simulink model "asbCubeSat"  (R2023b)
settings: Solver=FixedStepAuto  StartTime=0.0  StopTime=43200  FixedStep=CubeSatTimeStep  MaxStep=10  MinStep=0.01  RelTol=1e-7  AbsTol=1e-7  EnableMultiTasking=on
PreLoadFcn:
  | if ~builtin('license','test','Virtual_Reality_Toolbox')
  |     dd = Simulink.data.dictionary.open('asbCubeSatModelData.sldd');
  |     ddSect = getSection(dd, 'Design Data');
  |     assignin(ddSect,'variantVisualization',0)
  | end
InitFcn:
  | temp_dd = Simulink.data.dictionary.open('asbCubeSatModelData.sldd');
  | temp_ddSect = getSection(temp_dd, 'Design Data');
  | if evalin(temp_ddSect, 'variantVisualization == 1')
  |     if ~builtin('license','checkout','Virtual_Reality_Toolbox')
  |         error(message('aeroblks_cubesat:cubesat:licenseFailAnim'));
  |     end
  | end
  | clear temp_dd temp_ddSect;
undefined symbols (not defined in the file): actuator, asbCubeSatEnvironmentLib, CubeSatTimeStep, Enviroment, initCond, WMM2020
libraries: aerolibutil x16, sharedutil x4, aerolibconvert2 x4, matrix_library x3, aerolibattitudesys x2, simulink_extras x2, sharedtransform x2, aerolibgravity2 x1, SignalEditorBlockLib x1, aerolibtransform2 x1, asbCubeSatFSWLib x1, aerolibobsolete x1
settings Model: RequirementInfo={} %GIDa_aedc6be2_fb6a_446c_8c25_10b8bc9db182  DataDictionary=asbCubeSatModelData.sldd  SnapshotInterval=1  Creator=The MathWorks, Inc.  LastModifiedBy=Adin Sacho-Tanzer
settings SolverCC: AlgebraicLoopSolver=TrustRegion  MaxZcPerStep=1
settings DataIOCC: LimitDataPoints=on  SaveFormat=Array  SaveOutput=off  DSMLogging=off  SaveTime=off  ReturnWorkspaceOutputs=off
settings OptimizationCC: DefaultParameterBehavior=Inlined  OptimizeBlockIOStorage=off  BufferReuse=off  GlobalBufferReuse=off  ExpressionFolding=off  ExpressionDepthLimit=2147483647  LocalBlockOutputs=off  InitFltsAndDblsToZero=on  LifeSpan=inf  OptimizeDataStoreBuffers=off  BusAssignmentInplaceUpdate=off
settings DebuggingCC: SignalResolutionControl=TryResolveAllWithWarning  MultiTaskDSMMsg=warning  MultiTaskCondExecSysMsg=none  UnconnectedInputMsg=warning  UnconnectedOutputMsg=warning  UnconnectedLineMsg=warning  AssertControl=DisableAll  ModelReferenceExtraNoncontSigs=warning  StateNameClashWarn=warning  PregeneratedLibrarySubsystemCodeDiagnostic=none  SFUnexpectedBacktrackingDiag=warning  SFNoUnconditionalDefaultTransitionDiag=warning  SFExecutionAtInitializationDiag=none  ArithmeticOperatorsInVariantConditions=warning
settings HardwareCC: ProdBitPerPointer=32  ProdBitPerSizeT=32  ProdBitPerPtrDiffT=32  ProdLargestAtomicFloat=None  ProdIntDivRoundTo=Undefined  ProdEndianess=Unspecified  ProdWordSize=32  ProdHWDeviceType=32-bit Generic
settings ModelReferenceCC: UpdateModelReferenceTargets=IfOutOfDate  EnableRefExpFcnMdlSchedulingChecks=on  ModelReferenceMinAlgLoopOccurrences=on  PropagateSignalLabelsOutOfModel=off
settings SFSimCC: SimUseLocalCustomCode=off
settings RTWCC: RTWUseLocalCustomCode=off  DLArmComputeVersion=19.05
settings CodeAppCC: StateflowObjectComments=on
settings GRTTargetCC: TargetFcnLib=ansi_tfl_tmw.mat  TargetLangStandard=C89/C90 (ANSI)  CombineOutputUpdateFcns=off  GRTInterface=on
settings ConfigComp: CovMetricSettings=dw  CovSaveCumulativeToWorkspaceVar=on  CovSaveSingleToWorkspaceVar=on  CovExternalEMLEnable=off

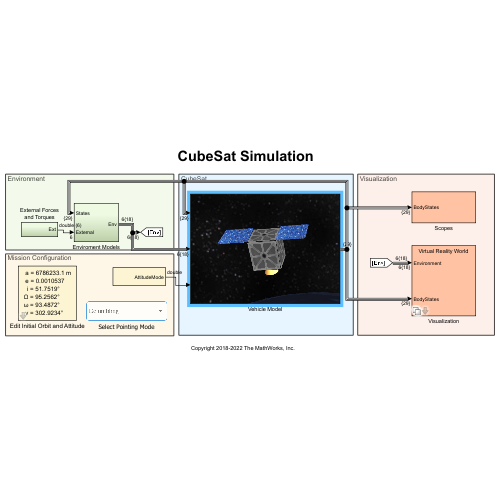
[thumbnail: Simulink's stored preview of the top-level diagram]
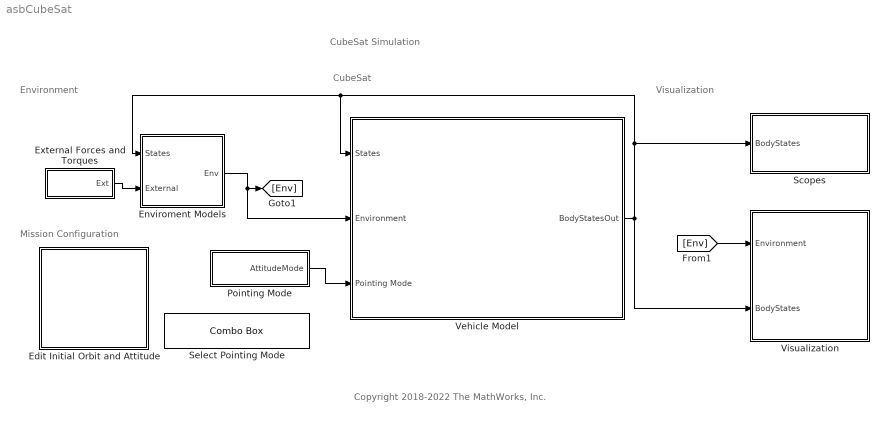
== system asbCubeSat ==
  note: Visualization
  note: CubeSat
  note: Environment
  note: Copyright 2018-2022 The MathWorks, Inc.
  note: CubeSat Simulation
  note: Mission Configuration
  Edit Initial Orbit and Attitude : Subsystem  mask(CubeSat Initial Conditions){sim_t0=2458488, epoch=2451545, method=Keplerian Orbital Elements, a=6786233.13, ecc=0.0010537, incl=51.7519, omega=95.2562, argp=93.4872, nu=302.9234, truelon=0, arglat=0, lonper=0, r_eci=[-2981784.257 5207055.9381 3161595.3068], v_eci=[-3384.4834 -4887.7595 4843.4609], r_ecef=[-5762650.9114 -1682704.282 3156028.2879], v_ecef=[3832.57 -4024.9014 4837.4311], lla=[27.88080034 -163.722102 408851.6223], v_ned=[5468.7396 4937.8129 -7.4627367], euler=[33.9 -5.91 9.88], pqr=[10 10 0]}
      mask prompts: sim_t0 "spacecraft:cubesat:StartDate"; epoch "spacecraft:cubesat:ECIEpoch"; method "spacecraft:cubesat:InputMethod"; a "spacecraft:cubesat:SemiMajorAxis"; ecc "spacecraft:cubesat:Eccentricity"; incl "spacecraft:cubesat:Inclination"; omega "spacecraft:cubesat:RAAN"; argp "spacecraft:cubesat:ArgP"; nu "spacecraft:cubesat:TrueAnomaly"; truelon "spacecraft:cubesat:TrueLon"; arglat "spacecraft:cubesat:ArgLat"; lonper "spacecraft:cubesat:LonPer"; r_eci "spacecraft:cubesat:ECIPos"; v_eci "spacecraft:cubesat:ECIVel"; r_ecef "spacecraft:cubesat:ECEFPos"; v_ecef "spacecraft:cubesat:ECEFVel"; lla "spacecraft:cubesat:LLA"; v_ned "spacecraft:cubesat:NEDVel"; euler "spacecraft:cubesat:Euler"; pqr "spacecraft:cubesat:BodyAngRates"
      mask help: spacecraft:cubesat:InitCondBlockDesc
      mask init:
      | initCond = cubeSatCallback(gcb, 'computeIC', method, sim_t0, epoch, a, ecc, incl,...
      |     omega, argp, nu, truelon, arglat, lonper, r_eci, v_eci, r_ecef, v_ecef, lla,...
      |     v_ned, euler, pqr);
      mask TypeOptions method: spacecraft:cubesat:InputKeplerian | spacecraft:cubesat:InputECI | spacecraft:cubesat:InputECEF | spacecraft:cubesat:InputLLANED
      mask Callback method: cubeSatCallback(gcb, 'handleMethod');
      mask Callback ecc: cubeSatCallback(gcb, 'handleCircularOrbit');
      mask Callback incl: cubeSatCallback(gcb, 'handleCircularOrbit');
      mask DialogControl sim_t0 Prompt: Start date [Julian date]:
      mask DialogControl sim_t0 Tooltip: spacecraft:spacecraft:StartDateTT
      mask DialogControl icTab Prompt: spacecraft:cubesat:InitCond
      mask DialogControl epoch Prompt: Epoch of ECI frame [Julian date]:
      mask DialogControl epoch Tooltip: spacecraft:cubesat:ECIEpochTT
      mask DialogControl Container9 Prompt: spacecraft:cubesat:InitCondOrbit
      mask DialogControl method Prompt: Input method:
      mask DialogControl method Tooltip: spacecraft:cubesat:InputMethodTT
      mask DialogControl a Prompt: Semi-major axis [m]:
      mask DialogControl a Tooltip: spacecraft:cubesat:SemiMajorAxisTT
      mask DialogControl ecc Prompt: Eccentricity:
      mask DialogControl ecc Tooltip: spacecraft:cubesat:EccentricityTT
      mask DialogControl incl Prompt: Inclination [deg]:
      mask DialogControl incl Tooltip: spacecraft:cubesat:InclinationTT
      mask DialogControl omega Prompt: Right ascension of the ascending node [deg]:
      mask DialogControl omega Tooltip: spacecraft:cubesat:RAANTT
      mask DialogControl argp Prompt: Argument of periapsis [deg]:
      mask DialogControl argp Tooltip: spacecraft:cubesat:ArgPTT
      mask DialogControl nu Prompt: True anomaly [deg]:
      mask DialogControl nu Tooltip: spacecraft:cubesat:TrueAnomalyTT
      mask DialogControl truelon Prompt: True longitude [deg] (circular equatorial):
      mask DialogControl truelon Tooltip: spacecraft:cubesat:TrueLonTT
      mask DialogControl arglat Prompt: Argument of latitude [deg] (circular inclined):
      mask DialogControl arglat Tooltip: spacecraft:cubesat:ArgLatTT
      mask DialogControl lonper Prompt: Longitude of periapsis [deg] (elliptical equatorial):
      mask DialogControl lonper Tooltip: spacecraft:cubesat:LonPerTT
      mask DialogControl r_eci Prompt: ECI position vector [m]:
      mask DialogControl r_eci Tooltip: spacecraft:cubesat:ECIPosTT
      mask DialogControl v_eci Prompt: ECI velocity vector [m/s]:
      mask DialogControl v_eci Tooltip: spacecraft:cubesat:ECIVelTT
      mask DialogControl r_ecef Prompt: ECEF position vector [m]:
      mask DialogControl r_ecef Tooltip: spacecraft:cubesat:ECEFPosTT
      mask DialogControl v_ecef Prompt: ECEF velocity vector [m/s]:
      mask DialogControl v_ecef Tooltip: spacecraft:cubesat:ECEFVelTT
      mask DialogControl lla Prompt: Geodetic latitude, longitude, altitude [deg, deg, m]:
      mask DialogControl lla Tooltip: spacecraft:cubesat:LLATT
      mask DialogControl v_ned Prompt: NED velocity vector [m/s]:
      mask DialogControl v_ned Tooltip: spacecraft:cubesat:NEDVelTT
      mask DialogControl Container11 Prompt: spacecraft:cubesat:InitCondAttitude
      mask DialogControl euler Prompt: Initial Euler angles (roll, pitch, yaw) [deg]:
      mask DialogControl euler Tooltip: spacecraft:cubesat:EulerTT
      mask DialogControl pqr Prompt: Initial body angular rates [deg/s]:
      mask DialogControl pqr Tooltip: spacecraft:cubesat:BodyAngRatesTT
      mask Display:
      | text(.1, .9, [' a = ' sprintf('%.1f', str2double(get_param(gcb, 'a'))) ' m'],'horizontalAlignment','left','texmode','on');
      | text(.1, .75, [' e = ' get_param(gcb, 'ecc')],'horizontalAlignment','left','texmode', 'on')
      | text(.1, .6, ['  i = ' get_param(gcb, 'incl') '\circ'],'horizontalAlignment','left','texmode', 'on')
      | text(.1, .45, ['\Omega = ' get_param(gcb, 'omega') '\circ'],'horizontalAlignment','left','texmode', 'on')
      | text(.1, .3, ['\omega = ' get_param(gcb, 'argp') '\circ'],'horizontalAlignment','left','texmode', 'on')
      | text(.1, .15, [' \nu = ' get_param(gcb, 'nu') '\circ'],'horizontalAlignment','left','texmode', 'on')
  Enviroment Models : Subsystem  AncestorBlock=asbCubeSatEnvironmentLib/Enviroment
  "External Forces and Torques " : Subsystem
  Pointing Mode : Subsystem
  Scopes : Subsystem  VariantControl=visOff
  Select Pointing Mode : ComboBox  LabelPosition=Hide  SelectedLabel=Detumbling
      settings: Values={{'Standby', 'Nadir Pointing (Earth)', 'Sun Tracking', 'Custom Schedule', 'Detumbling'}, [0 1 2 3 4]}
  Vehicle Model : Subsystem
      mask Display: image('CubeSatVehicle.PNG');
  Visualization : Subsystem  Variant=on  mask(Set Animation Properties){visSampleTime=5, cubesatSize=2e5, showAntenna=on, antennaHeight=1e6, antennaHalfAngle=25}
      mask prompts: visSampleTime "spacecraft:cubesat:AnimSampleTime"; cubesatSize "spacecraft:cubesat:MdlSize"; showAntenna "spacecraft:cubesat:ShowCone"; antennaHeight "spacecraft:cubesat:ConeHeight"; antennaHalfAngle "spacecraft:cubesat:ConeAngle"
      mask help: spacecraft:cubesat:VisBlockDesc
      mask Callback showAntenna:
      | if builtin('license','test','Virtual_Reality_Toolbox')
      | 
      |     enable = get_param(gcb,'MaskEnables');
      |     if strcmp(get_param(gcb, 'showAntenna'), 'off')
      |         enable(4:5) = {'off'};
      |     else
      |         enable(4:5) = {'on'};
      |     end
      |     set_param(gcb,'MaskEnables', enable);
      |     clear enable
      | end
      mask DialogControl vrOpenBtn Prompt: spacecraft:cubesat:AnimOpenBtn
      mask DialogControl vrOpenBtn Callback:
      | if builtin('license','checkout','Virtual_Reality_Toolbox')
      |     vrmfunc('FnOpen',getSimulinkBlockHandle([gcb '/Virtual Reality World/VR Sink']));
      | end
      mask DialogControl visSampleTime Prompt: Animation refresh rate:
      mask DialogControl visSampleTime Tooltip: spacecraft:cubesat:AnimSampleTimeTT
      mask DialogControl cubesatSize Prompt: CubeSat display size [m]:
      mask DialogControl cubesatSize Tooltip: spacecraft:cubesat:MdlSizeTT
      mask DialogControl Container3 Prompt: spacecraft:cubesat:AntennaPropArea
      mask DialogControl showAntenna Prompt: Show antenna cone in animation
      mask DialogControl showAntenna Tooltip: spacecraft:cubesat:ShowConeTT
      mask DialogControl antennaHeight Prompt: Antenna cone height [m]:
      mask DialogControl antennaHeight Tooltip: spacecraft:cubesat:ConeHeightTT
      mask DialogControl antennaHalfAngle Prompt: Antenna cone half angle [deg]:
      mask DialogControl antennaHalfAngle Tooltip: spacecraft:cubesat:ConeAngleTT
  wires:
  Enviroment Models/1(Env) -> Vehicle Model/2(Environment), [Env]
  "External Forces and Torques "/1(Ext) -> Enviroment Models/2(External)
  Pointing Mode/1(AttitudeMode) -> Vehicle Model/3(Pointing Mode)
  [Env] -> Visualization/1(Environment)
  Vehicle Model/1(BodyStatesOut) -> Visualization/2(BodyStates), Vehicle Model/1(States), Enviroment Models/1(States), Scopes/1(BodyStates)

== system asbCubeSat/Edit Initial Orbit and Attitude ==

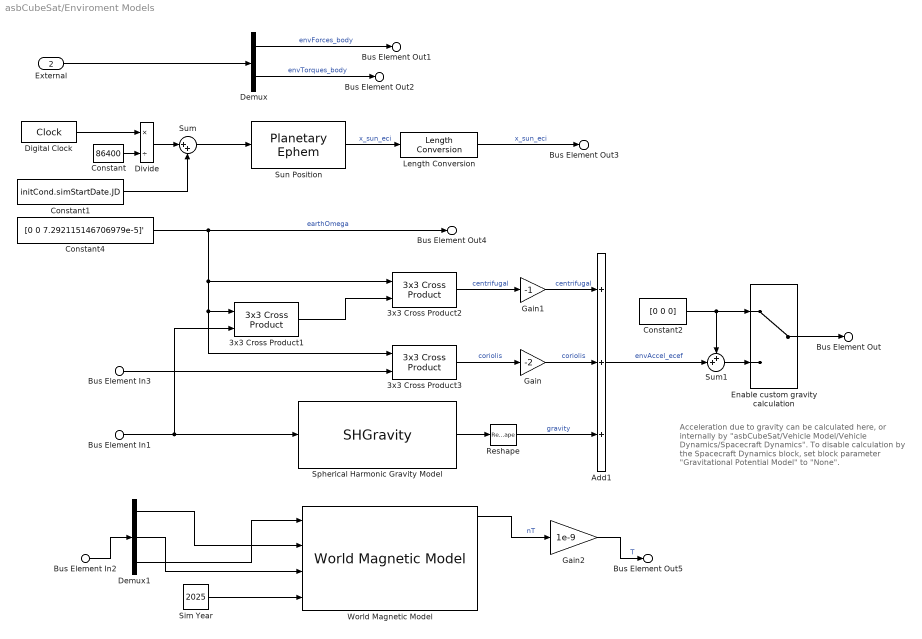
== system asbCubeSat/Enviroment Models ==
  note: Acceleration due to gravity can be calculated here, or internally by "asbCubeSat/Vehicle Model/Vehicle Dynamics/Spacecraft Dynamics". To disable calculation by the Spacecraft Dynamics block, set block parameter "Gravitational Potential Model" to "None".
  Bus Element In1 : Inport  PortName=States  Element=X_ecef
  Bus Element In3 : Inport  PortName=States  Element=V_ecef
  Bus Element In2 : Inport  PortName=States  Element=LatLonAlt
  External : Inport  RequirementInfo={} %GIDa_966e36cb_16b5_4872_900e_7ca1bd630c23  Port=2
  3x3 Cross Product1 : sharedutil/3x3 Cross Product  aMode=aMode
  3x3 Cross Product2 : sharedutil/3x3 Cross Product  aMode=aMode
  3x3 Cross Product3 : sharedutil/3x3 Cross Product  aMode=aMode
  Add1 : Sum  RequirementInfo={} %GIDa_b8d2c483_28a5_4509_a823_93e900185cc4  Inputs=+++
  Constant : Constant  Value=86400
  Constant1 : Constant  RequirementInfo={} %GIDa_d3dce1ea_7a4c_4489_9b49_860fce94c68a  Value=initCond.simStartDate.JD
  Constant2 : Constant  RequirementInfo={} %GIDa_bd077cfd_f306_41c3_b781_8f19467a1c05  Value=[0 0 0]
  Constant4 : Constant  Value=[0 0 7.292115146706979e-5]'
  Demux : Demux  RequirementInfo={} %GIDa_25e02362_af2f_4200_81e6_6d7271b48bfe  Outputs=2
  Demux1 : Demux  Outputs=3
  Digital Clock : DigitalClock  SampleTime=CubeSatTimeStep
  Divide : Product  Inputs=*/
  Enable custom gravity calculation : ManualSwitch
  Gain : Gain  Gain=-2
  Gain1 : Gain  Gain=-1
  Gain2 : Gain  Gain=1e-9
  Length Conversion : aerolibconvert2/Length Conversion  IU=km  OU=m
  Reshape : Reshape
  Sim Year : Constant  Value=2025
  Spherical Harmonic Gravity Model : SHGravity  RequirementInfo={} %GIDa_e6b23945_77d7_4eed_b23b_331bed44acc0  degree=20  datafile='aerogmm2b.mat'
  Sum : Sum  Inputs=|++
  Sum1 : Sum  Inputs=++|
  Sun Position : PlanetaryEphem  ephemerisModel=DE421  target=Sun  outputVelocity=off
  World Magnetic Model : aerolibgravity2/World Magnetic Model  model=WMM2020 (2020-2025)  customFile='WMM2020.COF'  units=Metric (MKS)  time_in=on  month=January  day=1  year=2020  action=Error  h_out=on  dec_out=on  inc_out=on  ti_out=on
  Bus Element Out : Outport  VectorParamsAs1DForOutWhenUnconnected=off  PortName=Env  Element=envAccel_ecef
  Bus Element Out1 : Outport  VectorParamsAs1DForOutWhenUnconnected=off  PortName=Env  Element=envForces_body
  Bus Element Out2 : Outport  VectorParamsAs1DForOutWhenUnconnected=off  PortName=Env  Element=envTorques_body
  Bus Element Out3 : Outport  VectorParamsAs1DForOutWhenUnconnected=off  PortName=Env  Element=x_sun_eci
  Bus Element Out4 : Outport  VectorParamsAs1DForOutWhenUnconnected=off  PortName=Env  Element=earthAngRate
  Bus Element Out5 : Outport  VectorParamsAs1DForOutWhenUnconnected=off  PortName=Env  Element=mag_NED
  wires:
  Sum1/1 -> Enable custom gravity calculation/2
  Enable custom gravity calculation/1 -> Bus Element Out/1
  Constant2/1 -> Enable custom gravity calculation/1, Sum1/1
  Gain/1 -> Add1/2  "coriolis"
  Gain1/1 -> Add1/1  "centrifugal"
  3x3 Cross Product2/1 -> Gain1/1  "centrifugal"
  3x3 Cross Product3/1 -> Gain/1  "coriolis"
  Bus Element In3/1 -> 3x3 Cross Product3/2
  3x3 Cross Product1/1 -> 3x3 Cross Product2/2
  Reshape/1 -> Add1/3  "gravity"
  Constant1/1 -> Sum/2
  Divide/1 -> Sum/1
  Constant/1 -> Divide/2
  Length Conversion/1 -> Bus Element Out3/1  "x_sun_eci"
  Constant4/1 -> 3x3 Cross Product2/1, 3x3 Cross Product1/1, 3x3 Cross Product3/1, Bus Element Out4/1  "earthOmega"
  Sun Position/1 -> Length Conversion/1  "x_sun_eci"
  Digital Clock/1 -> Divide/1
  Sum/1 -> Sun Position/1
  Spherical Harmonic Gravity Model/1 -> Reshape/1
  External/1 -> Demux/1
  Demux/2 -> Bus Element Out2/1  "envTorques_body"
  Add1/1 -> Sum1/2  "envAccel_ecef"
  Demux/1 -> Bus Element Out1/1  "envForces_body"
  Bus Element In1/1 -> Spherical Harmonic Gravity Model/1, 3x3 Cross Product1/2
  Bus Element In2/1 -> Demux1/1
  Demux1/1 -> World Magnetic Model/2
  Demux1/3 -> World Magnetic Model/1
  Demux1/2 -> World Magnetic Model/3
  Sim Year/1 -> World Magnetic Model/4
  World Magnetic Model/1 -> Gain2/1  "nT"
  Gain2/1 -> Bus Element Out5/1  "T"

== system asbCubeSat/External Forces and Torques  ==
  Forces_Body : Constant  Value=[0 0 0]
  Mux : Mux  RequirementInfo={} %GIDa_ef4ca723_4eef_40f8_bb1e_99de60d2b248  Inputs=2
  Torques_Body : Constant  Value=[0 0 0]
  Ext : Outport  RequirementInfo={} %GIDa_0f078eca_6127_499d_b81c_658503a40261  VectorParamsAs1DForOutWhenUnconnected=off
  wires:
  Forces_Body/1 -> Mux/1
  Torques_Body/1 -> Mux/2
  Mux/1 -> Ext/1

== system asbCubeSat/Pointing Mode ==
  note: Modes:
      | 0 = Off
      | 1 = Earth (Nadir)
      | 2 = Sun
  Mode : Constant  Value=4  SampleTime=-1
  Multiport Switch : MultiPortSwitch  DataPortOrder=Specify indices  DataPortIndices={3, [0,1,2]}  DiagnosticForDefault=None  SaturateOnIntegerOverflow=off  InputSameDT=off
  Signal Editor : SignalEditorBlockLib/Signal Editor  FileName=SignalEditorPointing.mat  ActiveScenario=PointingScenario  ActiveSignal=PointingMode  IsBus=off  OutputBusObjectStr=Bus: BusObject  SampleTime=0  Interpolate=off  ZeroCross=off  OutputAfterFinalValue=Setting to zero  Unit=inherit  PreserveSignalName=on  ApplySigPropsToAllScenarios=on  ApplySigPropsToAllSignals=off
  AttitudeMode : Outport  VectorParamsAs1DForOutWhenUnconnected=off
  wires:
  Signal Editor/1 -> Multiport Switch/2
  Mode/1 -> Multiport Switch/1, Multiport Switch/3
  Multiport Switch/1 -> AttitudeMode/1

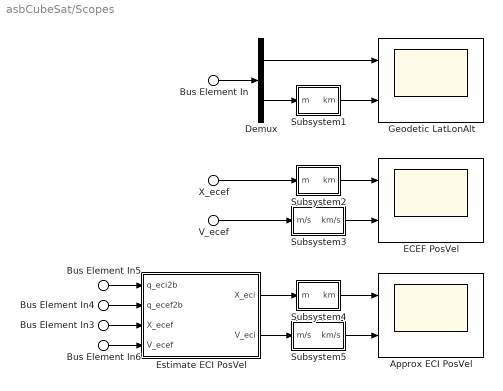
== system asbCubeSat/Scopes ==
  Bus Element In : Inport  PortName=BodyStates  Element=LatLonAlt
  X_ecef : Inport  PortName=BodyStates  Element=X_ecef
  Bus Element In3 : Inport  PortName=BodyStates  Element=X_ecef
  V_ecef : Inport  PortName=BodyStates  Element=V_ecef
  Bus Element In6 : Inport  PortName=BodyStates  Element=V_ecef
  Bus Element In4 : Inport  PortName=BodyStates  Element=q_ecef2b
  Bus Element In5 : Inport  PortName=BodyStates  Element=q_eci2b
  Approx ECI PosVel : Scope  NumInputPorts=2
  Demux : Demux  Outputs=[2 1]
  ECEF PosVel : Scope  NumInputPorts=2
  Estimate ECI PosVel : Subsystem
  Geodetic LatLonAlt : Scope  NumInputPorts=2
  Subsystem1 : Subsystem
  Subsystem2 : Subsystem
  Subsystem3 : Subsystem
  Subsystem4 : Subsystem
  Subsystem5 : Subsystem
  wires:
  Bus Element In/1 -> Demux/1
  Demux/1 -> Geodetic LatLonAlt/1
  Demux/2 -> Subsystem1/1(m)
  X_ecef/1 -> Subsystem2/1(m)
  V_ecef/1 -> Subsystem3/1(m/s)
  Estimate ECI PosVel/1(X_eci) -> Subsystem4/1(m)
  Estimate ECI PosVel/2(V_eci) -> Subsystem5/1(m/s)
  Bus Element In5/1 -> Estimate ECI PosVel/1(q_eci2b)
  Bus Element In4/1 -> Estimate ECI PosVel/2(q_ecef2b)
  Bus Element In3/1 -> Estimate ECI PosVel/3(X_ecef)
  Bus Element In6/1 -> Estimate ECI PosVel/4(V_ecef)
  Subsystem1/1(km) -> Geodetic LatLonAlt/2
  Subsystem2/1(km) -> ECEF PosVel/1
  Subsystem3/1(km/s) -> ECEF PosVel/2
  Subsystem4/1(km) -> Approx ECI PosVel/1
  Subsystem5/1(km/s) -> Approx ECI PosVel/2

== system asbCubeSat/Vehicle Model ==
  note: Flight Software
  note: Plant Model
  States : Inport
  Environment : Inport  Port=2
  Pointing Mode : Inport  Port=3
  Vehicle Control Actuators : Subsystem  AncestorBlock=asbCubeSatActuatorsLib/Vehicle Control Actuators
  Vehicle Control Sensors : Subsystem  AncestorBlock=asbCubeSatSensorsLib/Vehicle Control Sensors
  Vehicle Dynamics : Subsystem  AncestorBlock=asbCubeSatDynamicsLib/Vehicle Dynamics
  Vehicle Flight Software : asbCubeSatFSWLib/Vehicle Flight Software  SystemSampleTime=-1  VariantActivationTime=update diagram  AllowFlexibleInterface=on  Latency=0  AutoFrameSizeCalculation=off
  BodyStatesOut : Outport  OutDataTypeStr=Bus: StatesOutBus  VectorParamsAs1DForOutWhenUnconnected=off
  wires:
  Vehicle Dynamics/1(StatesOut) -> Vehicle Control Sensors/1(StatesOut), BodyStatesOut/1
  Pointing Mode/1 -> Vehicle Flight Software/1
  Vehicle Control Sensors/1(SensorsOut) -> Vehicle Flight Software/3
  Vehicle Control Actuators/1(" Forces") -> Vehicle Dynamics/1(Forces)
  Vehicle Control Actuators/2(" Torques") -> Vehicle Dynamics/2(Moments)
  Vehicle Flight Software/1 -> Vehicle Control Actuators/1(ActuatorCmds)
  Environment/1 -> Vehicle Control Actuators/2(Environment), Vehicle Dynamics/3(Env), Vehicle Flight Software/2
  States/1 -> Vehicle Control Actuators/3(States)

== system asbCubeSat/Visualization ==
  Environment : Inport
  BodyStates : Inport  RequirementInfo={} %GIDa_d1e0371a_f352_4707_a071_6ff04189e700  Port=2
  No Visualization : Subsystem  VariantControl=visOff
  Virtual Reality World : Subsystem  VariantControl=visSL3D

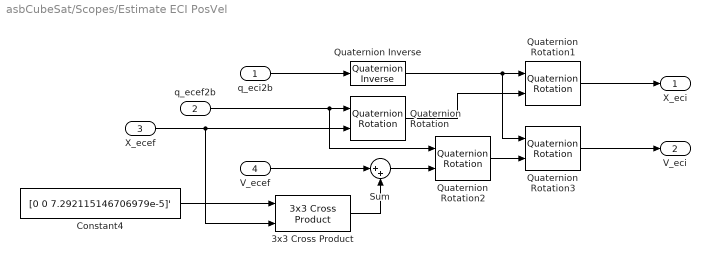
== system asbCubeSat/Scopes/Estimate ECI PosVel ==
  q_eci2b : Inport
  q_ecef2b : Inport  Port=2
  X_ecef : Inport  Port=3
  V_ecef : Inport  Port=4
  3x3 Cross Product : sharedutil/3x3 Cross Product  aMode=aMode
  Constant4 : Constant  Value=[0 0 7.292115146706979e-5]'
  Quaternion Inverse : aerolibutil/Quaternion Inverse
  Quaternion Rotation{,1..3} (4 alike) : aerolibutil/Quaternion Rotation
  Sum : Sum  Inputs=|++
  X_eci : Outport  VectorParamsAs1DForOutWhenUnconnected=off
  V_eci : Outport  Port=2  VectorParamsAs1DForOutWhenUnconnected=off
  wires:
  Sum/1 -> Quaternion Rotation2/2
  3x3 Cross Product/1 -> Sum/2
  V_ecef/1 -> Sum/1
  Quaternion Rotation/1 -> Quaternion Rotation1/2
  q_ecef2b/1 -> Quaternion Rotation/1, Quaternion Rotation2/1
  Quaternion Inverse/1 -> Quaternion Rotation3/1, Quaternion Rotation1/1
  Constant4/1 -> 3x3 Cross Product/1
  Quaternion Rotation2/1 -> Quaternion Rotation3/2
  q_eci2b/1 -> Quaternion Inverse/1
  Quaternion Rotation1/1 -> X_eci/1
  X_ecef/1 -> 3x3 Cross Product/2, Quaternion Rotation/2
  Quaternion Rotation3/1 -> V_eci/1

== system asbCubeSat/Scopes/Subsystem1 ==
  m : Inport  Unit=m
  Unit Conversion : UnitConversion
  km : Outport  Unit=km  VectorParamsAs1DForOutWhenUnconnected=off
  wires:
  m/1 -> Unit Conversion/1
  Unit Conversion/1 -> km/1

== system asbCubeSat/Scopes/Subsystem2 ==
  m : Inport  Unit=m
  Unit Conversion : UnitConversion
  km : Outport  Unit=km  VectorParamsAs1DForOutWhenUnconnected=off
  wires:
  Unit Conversion/1 -> km/1
  m/1 -> Unit Conversion/1

== system asbCubeSat/Scopes/Subsystem3 ==
  m/s : Inport  Unit=m/s
  Unit Conversion : UnitConversion
  km/s : Outport  Unit=km/s  VectorParamsAs1DForOutWhenUnconnected=off
  wires:
  m/s/1 -> Unit Conversion/1
  Unit Conversion/1 -> km/s/1

== system asbCubeSat/Scopes/Subsystem4 ==
  m : Inport  Unit=m
  Unit Conversion : UnitConversion
  km : Outport  Unit=km  VectorParamsAs1DForOutWhenUnconnected=off
  wires:
  Unit Conversion/1 -> km/1
  m/1 -> Unit Conversion/1

== system asbCubeSat/Scopes/Subsystem5 ==
  m/s : Inport  Unit=m/s
  Unit Conversion : UnitConversion
  km/s : Outport  Unit=km/s  VectorParamsAs1DForOutWhenUnconnected=off
  wires:
  m/s/1 -> Unit Conversion/1
  Unit Conversion/1 -> km/s/1

== system asbCubeSat/Vehicle Model/Vehicle Control Actuators ==
  ActuatorCmds : Inport  RequirementInfo={} %GIDa_020f38c4_9e26_4002_9065_5d46819fcfcb
  Environment : Inport  Port=2
  States : Inport  Port=3
  Magnetorquers : Subsystem  AncestorBlock=asbCubeSatActuatorsLib/CubeSat Perfect Actuators
  " Forces" : Outport  RequirementInfo={} %GIDa_e46e2c30_d205_4036_910c_a099c6c54d17  VectorParamsAs1DForOutWhenUnconnected=off
  " Torques" : Outport  RequirementInfo={} %GIDa_67b5453a_f72e_4aa8_be3c_a57a924d68da  Port=2  VectorParamsAs1DForOutWhenUnconnected=off
  wires:
  ActuatorCmds/1 -> Magnetorquers/1(ActuatorCmds)
  Environment/1 -> Magnetorquers/2(Environment)
  Magnetorquers/1(ForcesActual) -> " Forces"/1
  Magnetorquers/2(TorquesActual) -> " Torques"/1
  States/1 -> Magnetorquers/3(States)

== system asbCubeSat/Vehicle Model/Vehicle Control Sensors ==
  StatesOut : Inport  RequirementInfo={} %GIDa_90530906_86a2_4375_ad60_16b58fab3a32  OutDataTypeStr=Bus: StatesOutBus
  Unit Delay : UnitDelay  RequirementInfo={} %GIDa_09aaba6b_aadd_457c_a1ec_e9b9a273eb2e  Commented=through  SampleTime=CubeSatTimeStep  HasFrameUpgradeWarning=on
  SensorsOut : Outport  RequirementInfo={} %GIDa_3b6c2e72_aaee_4cf6_9430_15b046ac2608  OutDataTypeStr=Bus: StatesOutBus  VectorParamsAs1DForOutWhenUnconnected=off
  wires:
  Unit Delay/1 -> SensorsOut/1
  StatesOut/1 -> Unit Delay/1

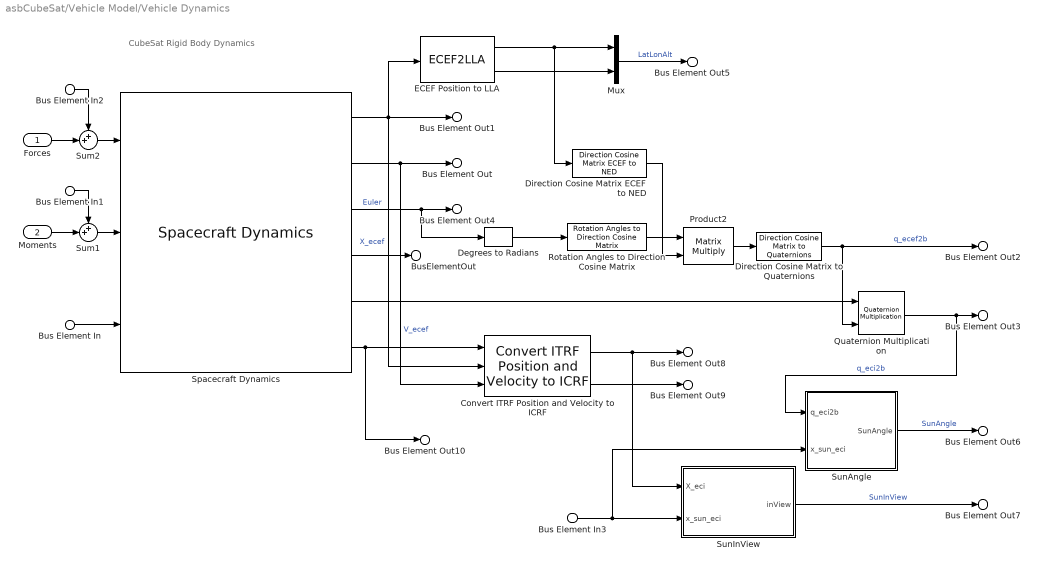
== system asbCubeSat/Vehicle Model/Vehicle Dynamics ==
  note: CubeSat Rigid Body Dynamics
  Forces : Inport  RequirementInfo={} %GIDa_ddd740cf_b998_4d50_bb9f_dead4dfb86ef
  Moments : Inport  RequirementInfo={} %GIDa_0e265085_ad05_44f5_915a_efdf50105eef  Port=2
  Bus Element In : Inport  Port=3  PortName=Env  Element=envAccel_ecef
  Bus Element In1 : Inport  Port=3  PortName=Env  Element=envTorques_body
  Bus Element In2 : Inport  Port=3  PortName=Env  Element=envForces_body
  Bus Element In3 : Inport  Port=3  PortName=Env  Element=x_sun_eci
  Convert ITRF Position and Velocity to ICRF : aerolibattitudesys/Convert ITRF Position and Velocity to ICRF
  Degrees to Radians : simulink_extras/Transformations/Degrees to Radians
  Direction Cosine Matrix ECEF to NED : aerolibtransform2/Direction Cosine Matrix ECEF to NED
  Direction Cosine Matrix to Quaternions : sharedtransform/Direction Cosine Matrix  to Quaternions  RequirementInfo={} %GIDa_3db19a8f_c925_4b51_9699_85867176506c  aMode=aMode  action=None  tolerance=eps(2)
  ECEF Position to LLA : ECEF2LLA
  Mux : Mux  Inputs=2
  Product2 : Product  Multiplication=Matrix(*)  RndMeth=Zero
  Quaternion Multiplication : aerolibutil/Quaternion Multiplication
  Rotation Angles to Direction Cosine Matrix : sharedtransform/Rotation Angles to Direction Cosine Matrix  rotationOrder=ZYX  aMode=aMode
  Spacecraft Dynamics : SpacecraftDynamics  accelIn=on  accelFrame=Fixed-frame  outportFrame=Fixed-frame  startDate=initCond.simStartDate.JD  mass=vehicle.mass  inertia=vehicle.inertia  stateFormatNum=ICRF state vector  inertialPosition=initCond.r_eci  inertialVelocity=initCond.v_eci  attitudeFrame=NED  attitudeFormat=Euler angles  attitude=initCond.euler  attitudeRate=initCond.pqr  outputTransform=on
  Sum1 : Sum  RequirementInfo={} %GIDa_57348fbd_ab1f_48c5_b399_5b65774ef7a8  Inputs=++|
  Sum2 : Sum  RequirementInfo={} %GIDa_1dfe2da7_e995_414b_aa51_4201cbd27953  Inputs=++|
  SunAngle : Subsystem
  SunInView : Subsystem
  Bus Element Out10 : Outport  VectorParamsAs1DForOutWhenUnconnected=off  PortName=StatesOut  Element=utc_JD
  Bus Element Out1 : Outport  VectorParamsAs1DForOutWhenUnconnected=off  PortName=StatesOut  Element=X_ecef
  Bus Element Out : Outport  VectorParamsAs1DForOutWhenUnconnected=off  PortName=StatesOut  Element=V_ecef
  Bus Element Out8 : Outport  VectorParamsAs1DForOutWhenUnconnected=off  PortName=StatesOut  Element=X_eci
  Bus Element Out9 : Outport  VectorParamsAs1DForOutWhenUnconnected=off  PortName=StatesOut  Element=V_eci
  Bus Element Out2 : Outport  VectorParamsAs1DForOutWhenUnconnected=off  PortName=StatesOut  Element=q_ecef2b
  Bus Element Out3 : Outport  VectorParamsAs1DForOutWhenUnconnected=off  PortName=StatesOut  Element=q_eci2b
  Bus Element Out4 : Outport  VectorParamsAs1DForOutWhenUnconnected=off  PortName=StatesOut  Element=Euler
  Bus Element Out5 : Outport  VectorParamsAs1DForOutWhenUnconnected=off  PortName=StatesOut  Element=LatLonAlt
  Bus Element Out6 : Outport  VectorParamsAs1DForOutWhenUnconnected=off  PortName=StatesOut  Element=SunAngle
  Bus Element Out7 : Outport  VectorParamsAs1DForOutWhenUnconnected=off  PortName=StatesOut  Element=SunInView
  BusElementOut : Outport  PortName=StatesOut  Element=omega_ned
  wires:
  Convert ITRF Position and Velocity to ICRF/2 -> Bus Element Out9/1
  Convert ITRF Position and Velocity to ICRF/1 -> SunInView/1(X_eci), Bus Element Out8/1
  SunInView/1(inView) -> Bus Element Out7/1  "SunInView"
  Bus Element In3/1 -> SunInView/2(x_sun_eci), SunAngle/2(x_sun_eci)
  SunAngle/1(SunAngle) -> Bus Element Out6/1  "SunAngle"
  Bus Element In2/1 -> Sum2/1
  Sum2/1 -> Spacecraft Dynamics/1
  Degrees to Radians/1 -> Rotation Angles to Direction Cosine Matrix/1
  Spacecraft Dynamics/6 -> Convert ITRF Position and Velocity to ICRF/1, Bus Element Out10/1
  Spacecraft Dynamics/4 -> BusElementOut/1
  Spacecraft Dynamics/5 -> Quaternion Multiplication/1
  Product2/1 -> Direction Cosine Matrix to Quaternions/1
  ECEF Position to LLA/1 -> Direction Cosine Matrix ECEF to NED/1, Mux/1
  Rotation Angles to Direction Cosine Matrix/1 -> Product2/1
  Direction Cosine Matrix ECEF to NED/1 -> Product2/2
  Spacecraft Dynamics/2 -> Convert ITRF Position and Velocity to ICRF/3, Bus Element Out/1  "V_ecef"
  Sum1/1 -> Spacecraft Dynamics/2
  Moments/1 -> Sum1/2
  Forces/1 -> Sum2/2
  Bus Element In/1 -> Spacecraft Dynamics/3
  Spacecraft Dynamics/3 -> Bus Element Out4/1, Degrees to Radians/1  "Euler"
  Mux/1 -> Bus Element Out5/1  "LatLonAlt"
  Direction Cosine Matrix to Quaternions/1 -> Quaternion Multiplication/2, Bus Element Out2/1  "q_ecef2b"
  Spacecraft Dynamics/1 -> ECEF Position to LLA/1, Convert ITRF Position and Velocity to ICRF/2, Bus Element Out1/1  "X_ecef"
  Bus Element In1/1 -> Sum1/1
  ECEF Position to LLA/2 -> Mux/2
  Quaternion Multiplication/1 -> Bus Element Out3/1, SunAngle/1(q_eci2b)  "q_eci2b"

== system asbCubeSat/Visualization/No Visualization ==
  BodyStates : Inport
  Environment : Inport  Port=2
  Terminator2 : Terminator
      settings: RequirementInfo={} %GIDa_803f6fff_5423_4e6f_a9df_7d3b0fb0a1d4
  Terminator3 : Terminator
      settings: RequirementInfo={} %GIDa_5d360e88_5b3d_45e7_ae99_5d46a57676c9
  wires:
  Environment/1 -> Terminator2/1
  BodyStates/1 -> Terminator3/1

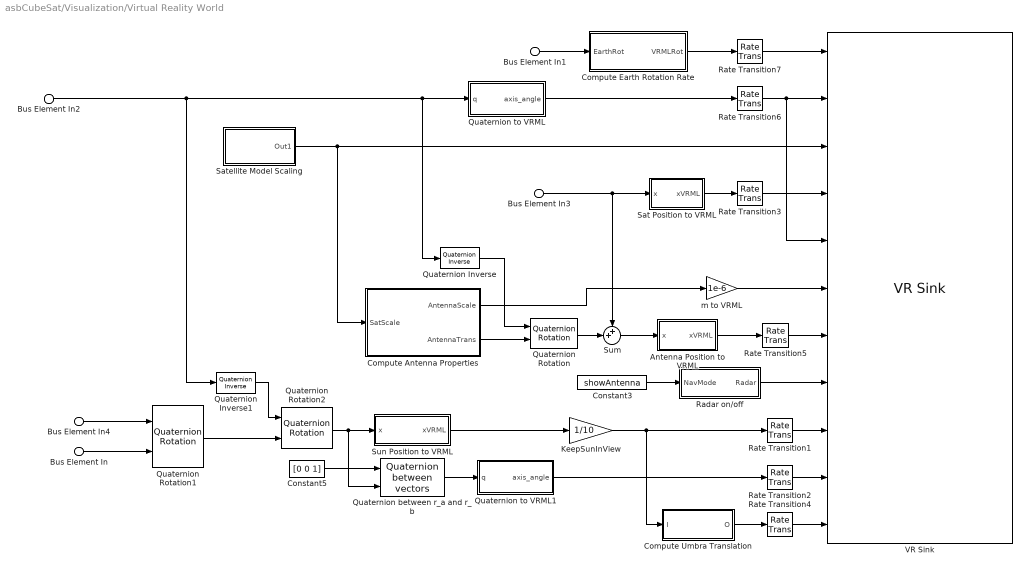
== system asbCubeSat/Visualization/Virtual Reality World ==
  Bus Element In3 : Inport  PortName=BodyStates  Element=X_ecef
  Bus Element In2 : Inport  PortName=BodyStates  Element=q_ecef2b
  Bus Element In4 : Inport  PortName=BodyStates  Element=q_eci2b
  Bus Element In : Inport  Port=2  PortName=Environment  Element=x_sun_eci
  Bus Element In1 : Inport  Port=2  PortName=Environment  Element=earthAngRate
  Antenna Position to VRML : Subsystem
  Compute Antenna Properties : Subsystem
  Compute Earth Rotation Rate : Subsystem
  Compute Umbra Translation : Subsystem
  Constant3 : Constant  Value=showAntenna
  Constant5 : Constant  Value=[0 0 1]
  KeepSunInView : Gain  Gain=1/10
  Quaternion Inverse : aerolibutil/Quaternion Inverse
  Quaternion Inverse1 : aerolibutil/Quaternion Inverse
  Quaternion Rotation : aerolibutil/Quaternion Rotation
  Quaternion Rotation1 : aerolibutil/Quaternion Rotation
  Quaternion Rotation2 : aerolibutil/Quaternion Rotation
  Quaternion between r_a and r_b : aerolibattitudesys/Quaternion between vectors
  Quaternion to VRML : Subsystem
  Quaternion to VRML1 : Subsystem
  Radar on/off : Subsystem
  Rate Transition{1..7} (7 alike) : RateTransition
  Sat Position to VRML : Subsystem
  Satellite Model Scaling : Subsystem
  Sum : Sum  Inputs=++|
  Sun Position to VRML : Subsystem
  VR Sink : vrlib/VR Sink  InstantiateOnLoad=on  SampleTime=visSampleTime  ViewEnable=on  RemoteChange=off  RemoteView=off  FieldsWritten=Earth.rotation.4.1.1.double#Satellite.rotation.4.1.1.double#Satellite.scale.3.1.1.double#Satellite.translation.3.1.1.double#AntennaCone.rotation.4.1.1.double#AntennaCone.scale.3.1.1.double#AntennaCone.translation.3.1.1.double#AntennaMaterial.transparency.1.1.1.double#Sun.translation.3.1.1.double#Umbra.rotation.4.1.1.double#Umbra.translation.3.1.1.double  WorldFileName=cubesatAnim.wrl  WorldDescription=CubeSat Orbit Animation  AutoView=on  VideoDimensions=[]  AllowVariableSize=off  FigureProperties="{'Position', 'Name', 'Viewpoint', 'CameraBound', 'CameraDirection', 'CameraPosition', 'CameraUpVector', 'ZoomFactor', 'Antialiasing', 'Headlight', 'Lighting', 'NavPanel', 'Sound', 'StatusBar', 'Stereo3D', 'Stereo3DCameraOffset', 'Stereo3DHIT', 'ToolBar', 'Textures', 'Transparency', 'Triad', 'Wireframe', 'NavZones', 'NavMode', 'NavSpeed', 'CaptureFileFormat', 'CaptureFileName', 'Record2DCompressMethod', 'Record2DCompressQuality', 'Record2D', 'Record2DFileName', 'Record2DFPS'; [5.0000000000000000e+00   9.2000000000000000e+01   5.7600000000000000e+02   3.5000000000000000e+02], 'CubeSat Orbit Animation', 'NorthPole', 'on', [0.0000000000000000e+00   0.0000000000000000e+00  -1.0000000000000000e+00], [0.0000000000000000e+00   0.0000000000000000e+00   0.0000000000000000e+00], [0.0000000000000000e+00   1.0000000000000000e+00   0.0000000000000000e+00], [1.0000000000000000e+00], 'on', 'on', 'on', 'halfbar', 'on', 'on', 'off', [1.0000000149011612e-01], [0.0000000000000000e+00], 'on', 'on', 'on', 'none', 'off', 'off', 'examine', 'normal', 'tif', '%f_anim_%n.tif', 'auto', [7.5000000000000000e+01], 'off', '%f_anim_%n.avi', 'auto'}"
  m to VRML : Gain  Gain=1e-6
  wires:
  Bus Element In2/1 -> Quaternion to VRML/1(q), Quaternion Inverse/1, Quaternion Inverse1/1
  Constant3/1 -> Radar on/off/1(NavMode)
  Bus Element In3/1 -> Sat Position to VRML/1(x), Sum/1
  Quaternion Inverse/1 -> Quaternion Rotation/1
  Sum/1 -> Antenna Position to VRML/1(x)
  Quaternion Rotation/1 -> Sum/2
  Quaternion Rotation2/1 -> Sun Position to VRML/1(x), Quaternion between r_a and r_b/2
  Quaternion Rotation1/1 -> Quaternion Rotation2/2
  Quaternion Inverse1/1 -> Quaternion Rotation2/1
  Sun Position to VRML/1(xVRML) -> KeepSunInView/1
  Quaternion between r_a and r_b/1 -> Quaternion to VRML1/1(q)
  Constant5/1 -> Quaternion between r_a and r_b/1
  m to VRML/1 -> VR Sink/6
  Antenna Position to VRML/1(xVRML) -> Rate Transition5/1
  Compute Earth Rotation Rate/1(VRMLRot) -> Rate Transition7/1
  Sat Position to VRML/1(xVRML) -> Rate Transition3/1
  Radar on/off/1(Radar) -> VR Sink/8
  Quaternion to VRML1/1(axis_angle) -> Rate Transition2/1
  KeepSunInView/1 -> Compute Umbra Translation/1(I), Rate Transition1/1
  Compute Umbra Translation/1(O) -> Rate Transition4/1
  Satellite Model Scaling/1(Out1) -> VR Sink/3, Compute Antenna Properties/1(SatScale)
  Compute Antenna Properties/1(AntennaScale) -> m to VRML/1
  Compute Antenna Properties/2(AntennaTrans) -> Quaternion Rotation/2
  Bus Element In4/1 -> Quaternion Rotation1/1
  Bus Element In/1 -> Quaternion Rotation1/2
  Rate Transition4/1 -> VR Sink/11
  Rate Transition1/1 -> VR Sink/9
  Rate Transition2/1 -> VR Sink/10
  Bus Element In1/1 -> Compute Earth Rotation Rate/1(EarthRot)
  Rate Transition7/1 -> VR Sink/1
  Rate Transition3/1 -> VR Sink/4
  Rate Transition5/1 -> VR Sink/7
  Quaternion to VRML/1(axis_angle) -> Rate Transition6/1
  Rate Transition6/1 -> VR Sink/5, VR Sink/2

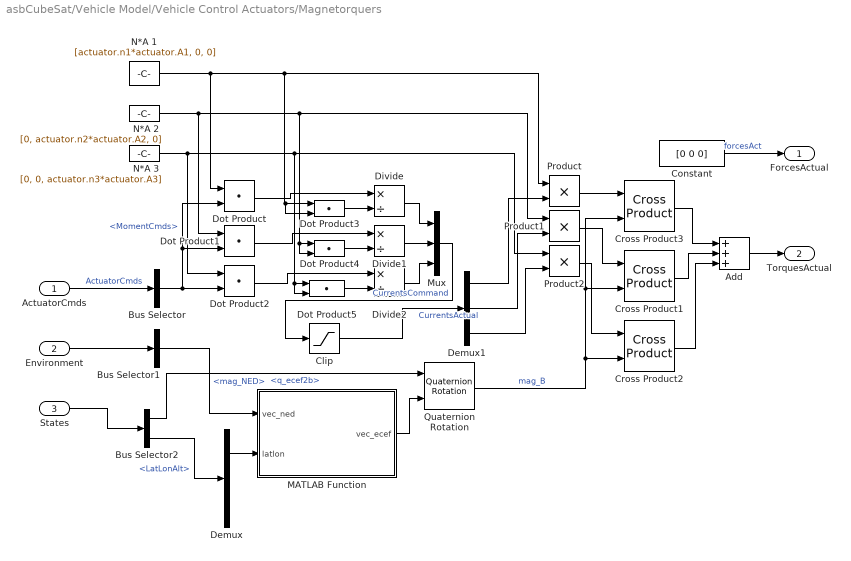
== system asbCubeSat/Vehicle Model/Vehicle Control Actuators/Magnetorquers ==
  ActuatorCmds : Inport  OutDataTypeStr=Bus: FCSOutBus
  Environment : Inport  Port=2
  States : Inport  Port=3
  Add : Sum  Inputs=+++
  Bus Selector : BusSelector  OutputSignals=ACSOut.MomentCmds
  Bus Selector1 : BusSelector  OutputSignals=mag_NED
  Bus Selector2 : BusSelector  OutputSignals=q_ecef2b,LatLonAlt
  Clip : Saturate  UpperLimit=actuator.maxCurrent  LowerLimit=-actuator.maxCurrent
  Constant : Constant  Value=[0 0 0]
  Cross Product1 : matrix_library/Cross Product
  Cross Product2 : matrix_library/Cross Product
  Cross Product3 : matrix_library/Cross Product
  Demux : Demux  Outputs=[2 1]
  Demux1 : Demux  Outputs=3
  Divide : Product  Inputs=*/
  Divide1 : Product  Inputs=*/
  Divide2 : Product  Inputs=*/
  Dot Product{,1..5} (6 alike) : DotProduct  OutDataTypeStr=Inherit: Inherit via internal rule
  MATLAB Function : MATLAB Function  TreatAsAtomicUnit=on
  Mux : Mux  Inputs=3
  N*A 1 : Constant  Value=[actuator.n1*actuator.A1, 0, 0]
  N*A 2 : Constant  Value=[0, actuator.n2*actuator.A2, 0]
  N*A 3 : Constant  Value=[0, 0, actuator.n3*actuator.A3]
  Product : Product
  Product1 : Product
  Product2 : Product
  Quaternion Rotation : aerolibutil/Quaternion Rotation
  ForcesActual : Outport  VectorParamsAs1DForOutWhenUnconnected=off
  TorquesActual : Outport  Port=2  VectorParamsAs1DForOutWhenUnconnected=off
  wires:
  Constant/1 -> ForcesActual/1  "forcesAct"
  ActuatorCmds/1 -> Bus Selector/1  "ActuatorCmds"
  Environment/1 -> Bus Selector1/1
  Bus Selector1/1 -> MATLAB Function/1(vec_ned)  "<mag_NED>"
  States/1 -> Bus Selector2/1
  Bus Selector2/2 -> Demux/1  "<LatLonAlt>"
  Demux/1 -> MATLAB Function/2(latlon)
  Bus Selector2/1 -> Quaternion Rotation/1  "<q_ecef2b>"
  MATLAB Function/1(vec_ecef) -> Quaternion Rotation/2
  Quaternion Rotation/1 -> Cross Product2/2, Cross Product1/2, Cross Product3/2  "mag_B"
  Clip/1 -> Demux1/1  "CurrentsActual"
  Demux1/1 -> Product/2
  N*A 1/1 -> Dot Product/1, Dot Product3/2, Dot Product3/1, Product/1
  N*A 2/1 -> Dot Product1/1, Dot Product4/2, Dot Product4/1, Product1/1
  N*A 3/1 -> Dot Product2/1, Dot Product5/2, Dot Product5/1, Product2/1
  Demux1/2 -> Product1/2
  Demux1/3 -> Product2/2
  Product/1 -> Cross Product3/1
  Product1/1 -> Cross Product1/1
  Product2/1 -> Cross Product2/1
  Cross Product3/1 -> Add/1
  Cross Product1/1 -> Add/2
  Cross Product2/1 -> Add/3
  Add/1 -> TorquesActual/1
  Mux/1 -> Clip/1  "CurrentsCommand"
  Bus Selector/1 -> Dot Product2/2, Dot Product/2, Dot Product1/2  "<MomentCmds>"
  Dot Product3/1 -> Divide/2
  Dot Product/1 -> Divide/1
  Dot Product1/1 -> Divide1/1
  Dot Product4/1 -> Divide1/2
  Dot Product5/1 -> Divide2/2
  Dot Product2/1 -> Divide2/1
  Divide/1 -> Mux/1
  Divide1/1 -> Mux/2
  Divide2/1 -> Mux/3

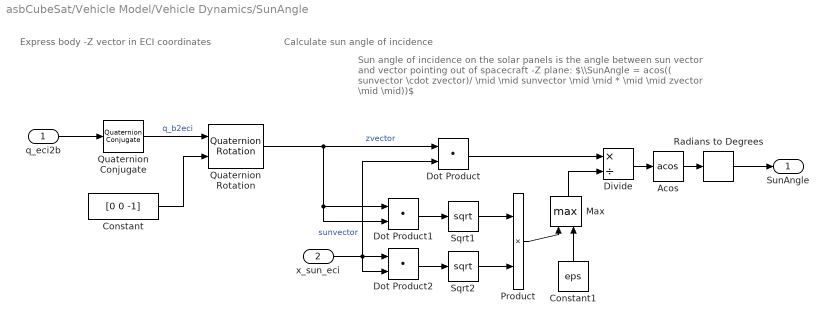
== system asbCubeSat/Vehicle Model/Vehicle Dynamics/SunAngle ==
  note: Sun angle of incidence on the solar panels is the angle between sun vector and vector pointing out of spacecraft -Z plane:
      | $\\SunAngle = acos(( sunvector \cdot zvector)/ \mid \mid sunvector \mid \mid * \mid \mid zvector \mid \mid))$
  note: Calculate sun angle of incidence
  note: Express body -Z vector in ECI coordinates
  q_eci2b : Inport  SampleTime=0
  x_sun_eci : Inport  Port=2  SampleTime=0
  Acos : Trigonometry  Operator=acos
  Constant : Constant  Value=[0 0 -1]  SampleTime=0
  Constant1 : Constant  Value=eps
  Divide : Product  Inputs=*/
  Dot Product : DotProduct  OutDataTypeStr=Inherit: Inherit via internal rule
  Dot Product1 : DotProduct  OutDataTypeStr=Inherit: Inherit via internal rule
  Dot Product2 : DotProduct  OutDataTypeStr=Inherit: Inherit via internal rule
  Max : MinMax  Function=max  Inputs=2
  Product : Product
  Quaternion Conjugate : aerolibutil/Quaternion Conjugate
  Quaternion Rotation : aerolibutil/Quaternion Rotation
  Radians to Degrees : simulink_extras/Transformations/Radians to Degrees
  Sqrt1 : Sqrt
  Sqrt2 : Sqrt
  SunAngle : Outport  SampleTime=0
  wires:
  Max/1 -> Divide/2
  Constant1/1 -> Max/2
  Product/1 -> Max/1
  Sqrt2/1 -> Product/2
  Sqrt1/1 -> Product/1
  Dot Product2/1 -> Sqrt2/1
  Quaternion Conjugate/1 -> Quaternion Rotation/1  "q_b2eci"
  q_eci2b/1 -> Quaternion Conjugate/1
  Constant/1 -> Quaternion Rotation/2
  Quaternion Rotation/1 -> Dot Product1/1, Dot Product1/2, Dot Product/1  "zvector"
  Dot Product1/1 -> Sqrt1/1
  Acos/1 -> Radians to Degrees/1
  Divide/1 -> Acos/1
  Dot Product/1 -> Divide/1
  x_sun_eci/1 -> Dot Product2/1, Dot Product2/2, Dot Product/2  "sunvector"
  Radians to Degrees/1 -> SunAngle/1

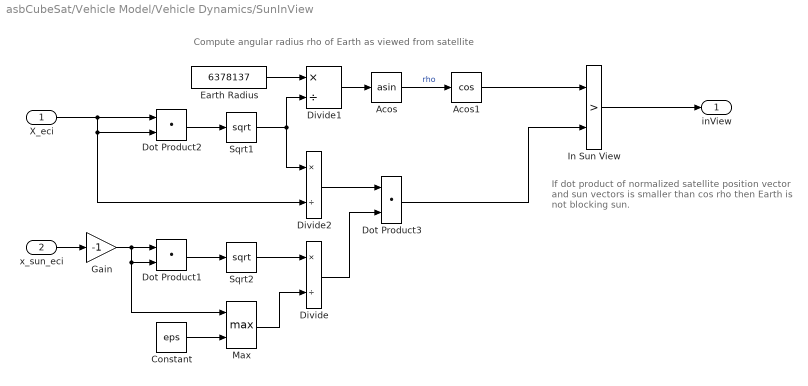
== system asbCubeSat/Vehicle Model/Vehicle Dynamics/SunInView ==
  note: If dot product of normalized satellite position vector and sun vectors is smaller than cos rho then Earth is not blocking sun.
  note: Compute angular radius rho of Earth as viewed from satellite
  X_eci : Inport
  x_sun_eci : Inport  Port=2  SampleTime=0
  Acos : Trigonometry  Operator=asin
  Acos1 : Trigonometry  Operator=cos
  Constant : Constant  Value=eps
  Divide : Product  Inputs=*/
  Divide1 : Product  Inputs=*/
  Divide2 : Product  Inputs=*/
  Dot Product1 : DotProduct  OutDataTypeStr=Inherit: Inherit via internal rule
  Dot Product2 : DotProduct  OutDataTypeStr=Inherit: Inherit via internal rule
  Dot Product3 : DotProduct  OutDataTypeStr=Inherit: Inherit via internal rule
  Earth Radius : Constant  Value=6378137  VectorParams1D=off  SampleTime=0
  Gain : Gain  Gain=-1
  In Sun View : RelationalOperator  Operator=>  OutDataTypeStr=boolean  ZeroCross=off  RndMeth=Simplest  InputSameDT=off
  Max : MinMax  Function=max  Inputs=2
  Sqrt1 : Sqrt
  Sqrt2 : Sqrt
  inView : Outport  SampleTime=0
  wires:
  Max/1 -> Divide/2
  Constant/1 -> Max/2
  Dot Product1/1 -> Sqrt2/1
  Sqrt2/1 -> Divide/1
  Dot Product3/1 -> In Sun View/2
  Divide2/1 -> Dot Product3/1
  Acos1/1 -> In Sun View/1
  Divide/1 -> Dot Product3/2
  Acos/1 -> Acos1/1  "rho"
  Divide1/1 -> Acos/1
  Sqrt1/1 -> Divide1/2, Divide2/1
  x_sun_eci/1 -> Gain/1
  Dot Product2/1 -> Sqrt1/1
  Earth Radius/1 -> Divide1/1
  X_eci/1 -> Dot Product2/1, Dot Product2/2, Divide2/2
  In Sun View/1 -> inView/1
  Gain/1 -> Dot Product1/1, Dot Product1/2, Max/1

== system asbCubeSat/Visualization/Virtual Reality World/Antenna Position to VRML ==
  x : Inport
  ECEF to VRML : Subsystem
  Length Conversion : aerolibconvert2/Length Conversion  IU=m  OU=km
  km to VRML units : Gain  Gain=1/1000
  xVRML : Outport  VectorParamsAs1DForOutWhenUnconnected=off
  wires:
  Length Conversion/1 -> km to VRML units/1
  km to VRML units/1 -> ECEF to VRML/1(M)
  x/1 -> Length Conversion/1
  ECEF to VRML/1(VR) -> xVRML/1

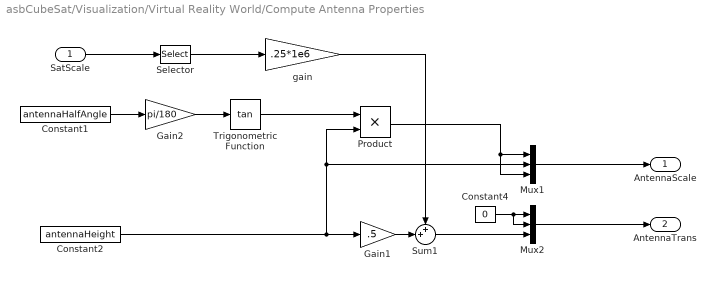
== system asbCubeSat/Visualization/Virtual Reality World/Compute Antenna Properties ==
  SatScale : Inport
  Constant1 : Constant  Value=antennaHalfAngle
  Constant2 : Constant  Value=antennaHeight
  Constant4 : Constant  Value=0
  Gain1 : Gain  Gain=.5
  Gain2 : Gain  Gain=pi/180
  Mux1 : Mux  Inputs=3
  Mux2 : Mux  Inputs=3
  Product : Product
  Selector : Selector  InputPortWidth=3  IndexOptions=Index vector (dialog)  Indices=1  OutputSizes=1
  Sum1 : Sum  Inputs=++|
  Trigonometric Function : Trigonometry  Operator=tan
  gain : Gain  Gain=.25*1e6
  AntennaScale : Outport  VectorParamsAs1DForOutWhenUnconnected=off
  AntennaTrans : Outport  Port=2  VectorParamsAs1DForOutWhenUnconnected=off
  wires:
  Gain2/1 -> Trigonometric Function/1
  Constant4/1 -> Mux2/1, Mux2/2
  Sum1/1 -> Mux2/3
  Constant2/1 -> Gain1/1, Mux1/2, Product/2
  gain/1 -> Sum1/1
  Constant1/1 -> Gain2/1
  Product/1 -> Mux1/3, Mux1/1
  Gain1/1 -> Sum1/2
  Trigonometric Function/1 -> Product/1
  Mux2/1 -> AntennaTrans/1
  Mux1/1 -> AntennaScale/1
  SatScale/1 -> Selector/1
  Selector/1 -> gain/1

== system asbCubeSat/Visualization/Virtual Reality World/Compute Earth Rotation Rate ==
  EarthRot : Inport
  Euler Angles to Quaternions : aerolibobsolete/Euler Angles to Quaternions
  Quaternion to VRML : Subsystem
  Sum : Sum  Inputs=|++
  Unit Delay : UnitDelay  SampleTime=-1  HasFrameUpgradeWarning=on
  VRMLRot : Outport  VectorParamsAs1DForOutWhenUnconnected=off
  wires:
  EarthRot/1 -> Sum/1
  Unit Delay/1 -> Sum/2
  Sum/1 -> Unit Delay/1, Euler Angles to Quaternions/1
  Euler Angles to Quaternions/1 -> Quaternion to VRML/1(q)
  Quaternion to VRML/1(AxisAngle) -> VRMLRot/1

== system asbCubeSat/Visualization/Virtual Reality World/Compute Umbra Translation ==
  I : Inport
  Add : Sum
  ConeHalfLength : Gain  Gain=692
  InvertSunPosECEF : Gain  Gain=-1
  unitVec : Subsystem
  O : Outport  VectorParamsAs1DForOutWhenUnconnected=off
  wires:
  ConeHalfLength/1 -> Add/2
  I/1 -> InvertSunPosECEF/1
  Add/1 -> O/1
  InvertSunPosECEF/1 -> unitVec/1(I), Add/1
  unitVec/1(O) -> ConeHalfLength/1

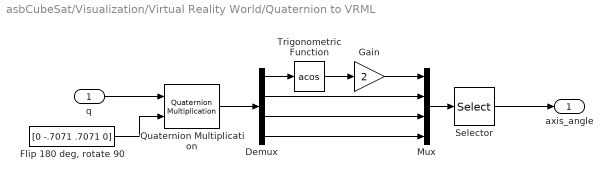
== system asbCubeSat/Visualization/Virtual Reality World/Quaternion to VRML ==
  q : Inport
  Demux : Demux
  "Flip 180 deg, rotate 90" : Constant  Value=[0 -.7071 .7071 0]
  Gain : Gain  Gain=2
  Mux : Mux
  Quaternion Multiplication : aerolibutil/Quaternion Multiplication
  Selector : Selector  InputPortWidth=4  IndexOptions=Index vector (dialog)  Indices=[3 4 2 1]  OutputSizes=1
  Trigonometric Function : Trigonometry  Operator=acos
  axis_angle : Outport  VectorParamsAs1DForOutWhenUnconnected=off
  wires:
  Demux/4 -> Mux/4
  Demux/3 -> Mux/3
  Demux/2 -> Mux/2
  Gain/1 -> Mux/1
  Selector/1 -> axis_angle/1
  q/1 -> Quaternion Multiplication/1
  Mux/1 -> Selector/1
  Trigonometric Function/1 -> Gain/1
  Demux/1 -> Trigonometric Function/1
  "Flip 180 deg, rotate 90"/1 -> Quaternion Multiplication/2
  Quaternion Multiplication/1 -> Demux/1

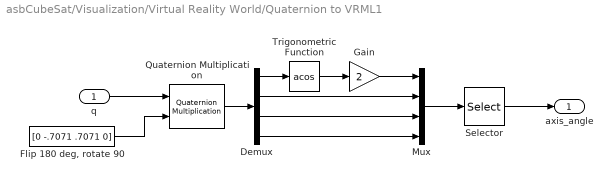
== system asbCubeSat/Visualization/Virtual Reality World/Quaternion to VRML1 ==
  q : Inport
  Demux : Demux
  "Flip 180 deg, rotate 90" : Constant  Value=[0 -.7071 .7071 0]
  Gain : Gain  Gain=2
  Mux : Mux
  Quaternion Multiplication : aerolibutil/Quaternion Multiplication
  Selector : Selector  InputPortWidth=4  IndexOptions=Index vector (dialog)  Indices=[3 4 2 1]  OutputSizes=1
  Trigonometric Function : Trigonometry  Operator=acos
  axis_angle : Outport  VectorParamsAs1DForOutWhenUnconnected=off
  wires:
  Demux/4 -> Mux/4
  Demux/3 -> Mux/3
  Demux/2 -> Mux/2
  Gain/1 -> Mux/1
  Selector/1 -> axis_angle/1
  Mux/1 -> Selector/1
  Trigonometric Function/1 -> Gain/1
  Demux/1 -> Trigonometric Function/1
  "Flip 180 deg, rotate 90"/1 -> Quaternion Multiplication/2
  q/1 -> Quaternion Multiplication/1
  Quaternion Multiplication/1 -> Demux/1

== system asbCubeSat/Visualization/Virtual Reality World/Radar on//off ==
  NavMode : Inport
  Add : Sum  Inputs=-+
  Compare To Constant : simulink/Logic and Bit Operations/Compare To Constant  relop===  const=1  OutDataTypeStr=boolean  ZeroCross=off
  Constant : Constant
  Data Type Conversion : DataTypeConversion  OutDataTypeStr=double  SaturateOnIntegerOverflow=off  RndMeth=Floor
  Gain : Gain  Gain=0.6
  Radar : Outport  VectorParamsAs1DForOutWhenUnconnected=off
  wires:
  NavMode/1 -> Compare To Constant/1
  Compare To Constant/1 -> Data Type Conversion/1
  Data Type Conversion/1 -> Gain/1
  Gain/1 -> Add/1
  Constant/1 -> Add/2
  Add/1 -> Radar/1

== system asbCubeSat/Visualization/Virtual Reality World/Sat Position to VRML ==
  x : Inport
  ECEF to VRML : Subsystem
  Length Conversion : aerolibconvert2/Length Conversion  IU=m  OU=km
  km to VRML units : Gain  Gain=1/1000
  xVRML : Outport  VectorParamsAs1DForOutWhenUnconnected=off
  wires:
  ECEF to VRML/1(VR) -> xVRML/1
  x/1 -> Length Conversion/1
  km to VRML units/1 -> ECEF to VRML/1(M)
  Length Conversion/1 -> km to VRML units/1

== system asbCubeSat/Visualization/Virtual Reality World/Satellite Model Scaling ==
  Constant : Constant  Value=cubesatSize
  Mux : Mux  Inputs=3
  ScaleModelToVRML : Gain  Gain=1/.3e6
  Out1 : Outport  VectorParamsAs1DForOutWhenUnconnected=off
  wires:
  ScaleModelToVRML/1 -> Mux/3, Mux/1, Mux/2
  Constant/1 -> ScaleModelToVRML/1
  Mux/1 -> Out1/1

== system asbCubeSat/Visualization/Virtual Reality World/Sun Position to VRML ==
  x : Inport
  ECEF to VRML : Subsystem
  Length Conversion : aerolibconvert2/Length Conversion  IU=m  OU=km
  km to VRML units : Gain  Gain=1/1000
  xVRML : Outport  VectorParamsAs1DForOutWhenUnconnected=off
  wires:
  ECEF to VRML/1(VR) -> xVRML/1
  x/1 -> Length Conversion/1
  km to VRML units/1 -> ECEF to VRML/1(M)
  Length Conversion/1 -> km to VRML units/1

== system asbCubeSat/Visualization/Virtual Reality World/Antenna Position to VRML/ECEF to VRML ==
  M : Inport  PortDimensions=3
  Selector : Selector  InputPortWidth=3  IndexOptions=Index vector (dialog)  Indices=[2 3 1]  OutputSizes=1
  VR : Outport  PortDimensions=3  VectorParamsAs1DForOutWhenUnconnected=off
  wires:
  M/1 -> Selector/1
  Selector/1 -> VR/1

== system asbCubeSat/Visualization/Virtual Reality World/Compute Earth Rotation Rate/Quaternion to VRML ==
  q : Inport
  Demux : Demux
  Gain : Gain  Gain=2
  Gain3 : Gain  Gain=[-1 1 1 1]
  Mux : Mux
  Selector : Selector  InputPortWidth=4  IndexOptions=Index vector (dialog)  Indices=[2 4 3 1]  OutputSizes=1
  Trigonometric Function : Trigonometry  Operator=acos
  AxisAngle : Outport  VectorParamsAs1DForOutWhenUnconnected=off
  wires:
  Demux/4 -> Mux/4
  Demux/3 -> Mux/3
  Demux/2 -> Mux/2
  Gain/1 -> Mux/1
  Selector/1 -> Gain3/1
  Gain3/1 -> AxisAngle/1
  q/1 -> Demux/1
  Mux/1 -> Selector/1
  Trigonometric Function/1 -> Gain/1
  Demux/1 -> Trigonometric Function/1

== system asbCubeSat/Visualization/Virtual Reality World/Compute Umbra Translation/unitVec ==
  I : Inport
  Divide : Product  Inputs=*/
  Dot Product : DotProduct  OutDataTypeStr=Inherit: Inherit via internal rule
  Sqrt : Sqrt
  O : Outport  VectorParamsAs1DForOutWhenUnconnected=off
  wires:
  Dot Product/1 -> Sqrt/1
  I/1 -> Divide/1, Dot Product/1, Dot Product/2
  Divide/1 -> O/1
  Sqrt/1 -> Divide/2

== system asbCubeSat/Visualization/Virtual Reality World/Sat Position to VRML/ECEF to VRML ==
  M : Inport  PortDimensions=3
  Selector : Selector  InputPortWidth=3  IndexOptions=Index vector (dialog)  Indices=[2 3 1]  OutputSizes=1
  VR : Outport  PortDimensions=3  VectorParamsAs1DForOutWhenUnconnected=off
  wires:
  M/1 -> Selector/1
  Selector/1 -> VR/1

== system asbCubeSat/Visualization/Virtual Reality World/Sun Position to VRML/ECEF to VRML ==
  M : Inport  PortDimensions=3
  Selector : Selector  InputPortWidth=3  IndexOptions=Index vector (dialog)  Indices=[2 3 1]  OutputSizes=1
  VR : Outport  PortDimensions=3  VectorParamsAs1DForOutWhenUnconnected=off
  wires:
  M/1 -> Selector/1
  Selector/1 -> VR/1

== matlab function asbCubeSat/Vehicle Model/Vehicle Control Actuators/Magnetorquers/MATLAB Function ==
  data: vec_ned input; vec_ecef output double size=[3 1]; latlon input
function vec_ecef = convert_ned2ecef(vec_ned, latlon)

vec_ecef = zeros(3,1);

uN = vec_ned(1);
vE = vec_ned(2);
wD = vec_ned(3);

lat = deg2rad(latlon(1));
lon = deg2rad(latlon(2));

sLat = sin(lat);
cLat = cos(lat);
sLon = sin(lon);
cLon = cos(lon);

vec_ecef(1) = -sLat*cLon*uN - sLon*vE - cLat*cLon*wD;
vec_ecef(2) = -sLat*sLon*uN + cLon*vE - cLat*sLon*wD;
vec_ecef(3) =  cLat*uN              - sLat*wD;

end
